simulink model "sampleModel340"  (R2021b)
settings: Solver=VariableStepAuto  StartTime=0.0  StopTime=10.0  RelTol=1e-3
libraries: simulink x2
settings Model: Creator=user  LastModifiedBy=user

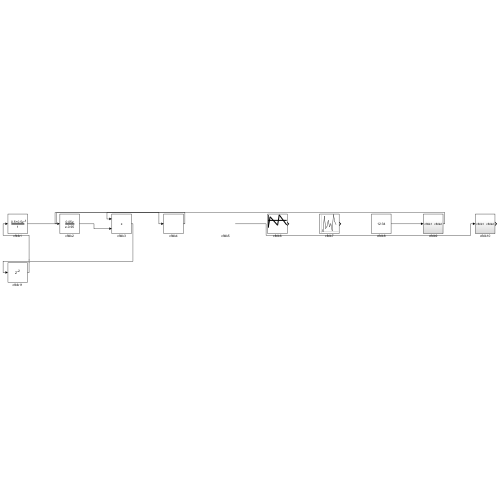
[thumbnail: Simulink's stored preview of the top-level diagram]
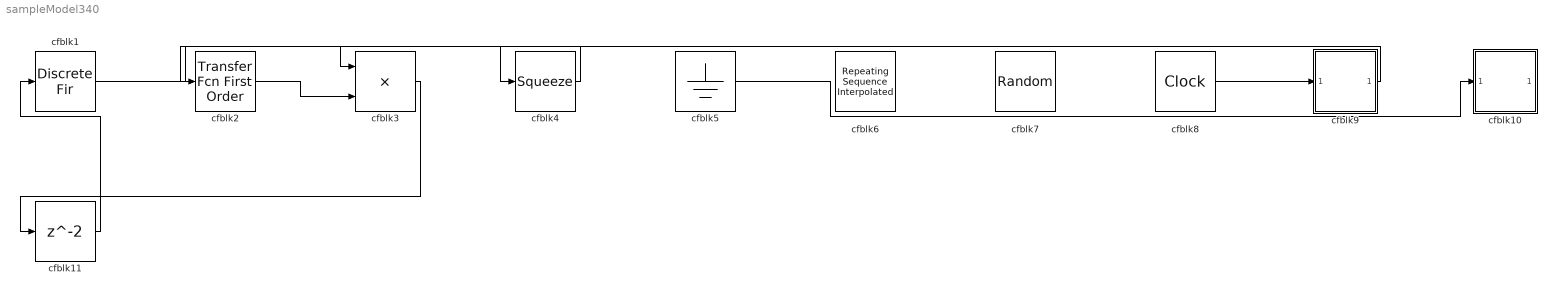
== system sampleModel340 ==
  cfblk1 : DiscreteFir  SampleTime=1
  cfblk10 : Subsystem
  cfblk11 : Delay  SampleTime=1
  cfblk2 : simulink/Discrete/Transfer Fcn First Order  PoleZ=0.95  ICPrevOutput=0.0  DoSatur=off
  cfblk3 : Product
  cfblk4 : Squeeze
  cfblk5 : Ground
  cfblk6 : simulink/Sources/Repeating Sequence Interpolated  OutValues=[-929896268.538464, 436045635.665129, -653621899.387239, 705900682.167253, -614373188.256633]  TimeValues=[0 0.1 0.5 0.6 1].'  LookUpMeth=Use Input Below  tsamp=0.01  OutMin=[]  OutMax=[]  OutDataTypeStr=double  OutputDataTypeScalingMode=double  OutDataType=fixdt(0,8)  OutScaling=2^-10
  cfblk7 : UniformRandomNumber  Minimum=[-9371029914.599783]  Maximum=[532665975.214297]  Seed=[67591967.000000]  SampleTime=0.1
  cfblk8 : DigitalClock
  cfblk9 : Subsystem
  wires:
  cfblk8/1 -> cfblk9/1(cfblk1)
  cfblk9/1(cfblk2) -> cfblk3/1
  cfblk2/1 -> cfblk3/2
  cfblk1/1 -> cfblk4/1
  cfblk4/1 -> cfblk2/1
  cfblk5/1 -> cfblk10/1(cfblk1)
  cfblk3/1 -> cfblk11/1
  cfblk11/1 -> cfblk1/1

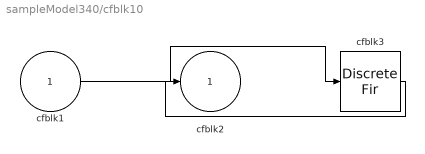
== system sampleModel340/cfblk10 ==
  cfblk1 : Inport
  cfblk3 : DiscreteFir  SampleTime=1
  cfblk2 : Outport
  wires:
  cfblk1/1 -> cfblk3/1
  cfblk3/1 -> cfblk2/1

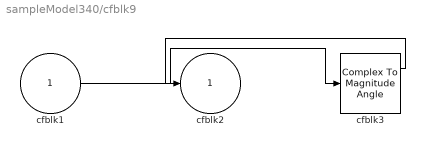
== system sampleModel340/cfblk9 ==
  cfblk1 : Inport
  cfblk3 : ComplexToMagnitudeAngle
  cfblk2 : Outport
  wires:
  cfblk1/1 -> cfblk3/1
  cfblk3/1 -> cfblk2/1
